simulink model "x8DOF_Robot"  (R2021a)
settings: Solver=FixedStepAuto  StartTime=0.0  StopTime=inf  RelTol=1e-3
InitFcn:
  | addpath("8DOF_robotModel\robot\")
  | run("x8DOF_Robot_DataFile.m")
model workspace: external: MATLAB File U:\Stage\8D-LMPM_Main\8D-LMPM_Matlab_Functions\8DOF_robotModel\x8DOF_Robot_DataFile.m (data not in the file)
values from neighbouring files (symbols this model uses):
  smiData = struct    [x8DOF_Robot_DataFile.m]
undefined symbols (not defined in the file or in its folder): rho_Command, X, Y, Z
libraries: sm_lib x422, nesl_utility x14
(part 1 of 8)
settings Model: OrderedModelArguments=off  Creator=MNLER  LastModifiedBy=MNLER
settings ExplorerConfigSet: InternalSimMechanicsExplorerSettings="<ExplorerConfiguration><canonicalview>default</canonicalview><AnimationSetting><BasePlaybackSpeed>1.0</BasePlaybackSpeed><PlaybackSpeedFactor>128.0</PlaybackSpeedFactor></AnimationSetting><TilePanel><TileInfo><Tiles Columns=\"1\" Count=\"1\" Rows=\"1\"><Column Weight=\"1\"/><Row Weight=\"1\"/><Tile Height=\"1\" Width=\"1\" X=\"0\" Y=\"0\"/></Tiles></TileInfo><SceneInfo><SceneViewer><BGColor><R>0.60000002384185791</R><G>0.60000002384185791</G><B>0.60000002384185791</B></BGColor><Camera><DoPerspective>off</DoPerspective><Position><X>0.435748104346844967</X><Y>-0.946733489107650761</Y><Z>-0.270829319928131862</Z></Position><Center><X>0.0638796881970406516</X><Y>-0.0352576872874645897</Y><Z>-0.446686488581036767</Z></Center><Up><X>0.0418696917330604879</X><Y>0.205719334419891764</Y><Z>0.977714930007727578</Z></Up><ViewLimDist>1</ViewLimDist><YLim>0.297781951931052613</YLim><XLim>0.45105207424850613</XLim></Camera></SceneViewer></SceneInfo></TilePanel><MechEditorPanel><Cameras/><GfxPanelCameraMap/><VideoCreator><PlaybackSpeedRatio>1.0</PlaybackSpeedRatio><FrameRate>30</FrameRate><VideoFormat>Motion JPEG AVI</VideoFormat><FrameSize>auto</FrameSize></VideoCreator></MechEditorPanel></ExplorerConfiguration>"

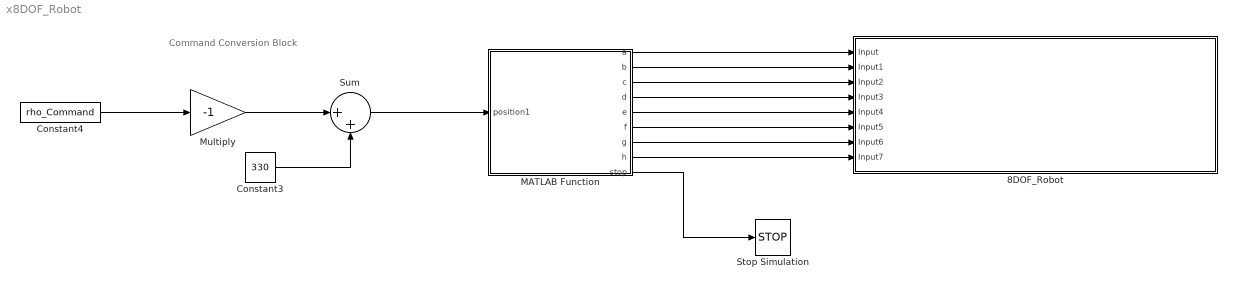
== system x8DOF_Robot ==
  note: Command Conversion Block
  8DOF_Robot : Subsystem
  Constant3 : Constant  Value=330
  Constant4 : Constant  Value=rho_Command
  MATLAB Function : MATLAB Function  TreatAsAtomicUnit=on
  Multiply : Gain  Gain=-1
  Stop Simulation : Stop
  Sum : Sum  Inputs=|++
  wires:
  MATLAB Function/1(a) -> 8DOF_Robot/1(Input)
  MATLAB Function/2(b) -> 8DOF_Robot/2(Input1)
  MATLAB Function/3(c) -> 8DOF_Robot/3(Input2)
  MATLAB Function/4(d) -> 8DOF_Robot/4(Input3)
  MATLAB Function/5(e) -> 8DOF_Robot/5(Input4)
  MATLAB Function/6(f) -> 8DOF_Robot/6(Input5)
  MATLAB Function/7(g) -> 8DOF_Robot/7(Input6)
  MATLAB Function/8(h) -> 8DOF_Robot/8(Input7)
  MATLAB Function/9(stop) -> Stop Simulation/1
  Multiply/1 -> Sum/1
  Sum/1 -> MATLAB Function/1(position1)
  Constant3/1 -> Sum/2
  Constant4/1 -> Multiply/1
